simulink model "pdmTransmissionCasing3_new"  (R2020b)
settings: Solver=VariableStepAuto  StartTime=0.0  StopTime=50  FixedStep=0.1  MaxStep=1e-1  RelTol=1e-1  AbsTol=1e-1  EnableMultiTasking=on
PreLoadFcn:
  | ClutchRadius = 100;
  | DampingCoeff = 0.1;
  | SGain = 1;
  | ShaftWear = 0;
  | ToothFaultGain = 0;
  | SDrift = 0;
undefined symbols (not defined in the file or in its folder): sigbuilder_block
libraries: fl_lib x42, nesl_utility x22, sdl_lib x6, commchan3 x2
(part 2 of 2)

== matlab function pdmTransmissionCasing3_new/AMPRBS DRIVE TORQUE/Amplitude Modulated Pseudo-Random Bit Sequences ==
  data: time input; min_hold_time input; max_hold_time input; min_value input; max_value input; random_value input; random_value output; random_hold_time input; random_hold_time output; previous_holding_time input; previous_holding_time output
function [random_value, random_hold_time, previous_holding_time]= fcn(time, min_hold_time, max_hold_time, min_value, max_value, random_value, random_hold_time, previous_holding_time)
%to reseeds the generator
if previous_holding_time + random_hold_time <= time
    rng('shuffle')
    random_value = (max_value-min_value)*rand(1,1) + min_value;
    random_hold_time = (max_hold_time - min_hold_time)*rand(1,1) + min_hold_time;
    previous_holding_time = time;
end

== matlab function pdmTransmissionCasing3_new/AMPRBS GEAR/Amplitude Modulated Pseudo-Random Bit Sequences ==
  data: time input; min_hold_time input; max_hold_time input; min_value input; max_value input; int_value input; random_value input; random_value output; random_hold_time input; random_hold_time output; previous_holding_time input; previous_holding_time output
function [random_value, random_hold_time, previous_holding_time]= fcn(time, min_hold_time, max_hold_time, min_value, max_value, int_value, random_value, random_hold_time, previous_holding_time)
%#codegen
if previous_holding_time + random_hold_time <= time
    %zmiana ziarna zeby inne losowanie za kazdym razem bylo
    rng('shuffle')
    %jezeli int_value = 1 to losuj tylko calkowite liczby z zakresu w
    %przeciwnym razie tez niecalkowite
    if int_value == 1 
        random_value = randi([min_value max_value]);
    else
        random_value = (max_value-min_value)*rand(1,1) + min_value;
    end
    random_hold_time = (max_hold_time - min_hold_time)*rand(1,1) + min_hold_time;
    previous_holding_time = time;
end

== matlab function pdmTransmissionCasing3_new/Tacho Sensor/Tacho sensor ==
  data: u input; previous_catch input; full_turn output; new_catch output
function [full_turn, new_catch]= fcn(u, previous_catch)
%to reseeds the generator
full_turn = 0;
new_catch = previous_catch;
if abs(previous_catch - u) >= 2 * pi
    full_turn = 1;
    new_catch =u; 
end

== matlab function pdmTransmissionCasing3_new/Tacho Sensor/Tacho sensor1 ==
  data: u input; previous_catch input; full_turn output; new_catch output
function [full_turn, new_catch]= fcn(u, previous_catch)
%to reseeds the generator
full_turn = 0;
new_catch = previous_catch;
if abs(previous_catch - u) >= 2 * pi
    full_turn = 1;
    new_catch =u; 
end

== matlab function pdmTransmissionCasing3_new/Tacho Sensor/Tacho sensor2 ==
  data: u input; previous_catch input; full_turn output; new_catch output
function [full_turn, new_catch]= fcn(u, previous_catch)
%to reseeds the generator
full_turn = 0;
new_catch = previous_catch;
if abs(previous_catch - u) >= 2 * pi
    full_turn = 1;
    new_catch =u; 
end
